simulink model "motor_final"  (R2019a)
settings: Solver=VariableStepAuto  StartTime=0.0  StopTime=10.0  RelTol=1e-3
values from neighbouring files (symbols this model uses):
  B = .1    (= 0.1)    [parameters.m]
  J = .01    (= 0.01)    [parameters.m]
  K = .01    (= 0.01)    [parameters.m]
  L = .5    (= 0.5)    [parameters.m]
  R = 1    [parameters.m]
settings Model: Creator=Victor  LastModifiedBy=Victor

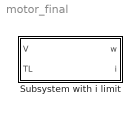
== system motor_final ==
  Subsystem with i limit : Subsystem

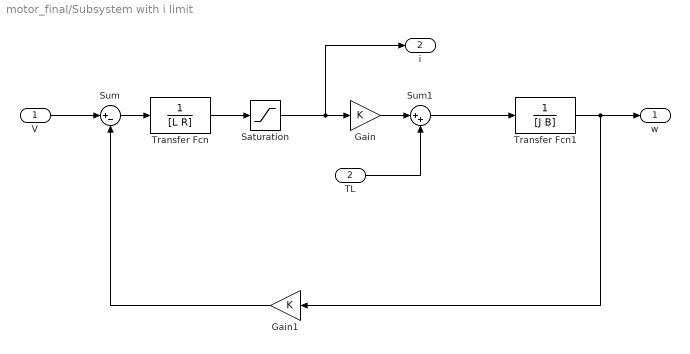
== system motor_final/Subsystem with i limit ==
  V : Inport
  TL : Inport  Port=2
  Gain : Gain  Gain=K
  Gain1 : Gain  Gain=K
  Saturation : Saturate  UpperLimit=20  LowerLimit=-20
  Sum : Sum  Inputs=|+-
  Sum1 : Sum  Inputs=|++
  Transfer Fcn : TransferFcn  Denominator=[L R]
  Transfer Fcn1 : TransferFcn  Denominator=[J B]
  w : Outport
  i : Outport  Port=2
  wires:
  Transfer Fcn1/1 -> w/1, Gain1/1
  Gain1/1 -> Sum/2
  V/1 -> Sum/1
  Sum/1 -> Transfer Fcn/1
  Transfer Fcn/1 -> Saturation/1
  Gain/1 -> Sum1/1
  Sum1/1 -> Transfer Fcn1/1
  TL/1 -> Sum1/2
  Saturation/1 -> Gain/1, i/1
